simulink model "traj_generator"  (R2020b)
settings: Solver=ode45  StartTime=0.0  StopTime=1  MaxStep=0.01  RelTol=1e-3
values from neighbouring files (symbols this model uses):
  g = 9.81    [matlab.mat]
  m = 1.5    [matlab.mat]
undefined symbols (not defined in the file or in its folder): k_Y, x_dot_min
settings Model: Creator=Danil  LastModifiedBy=Danil

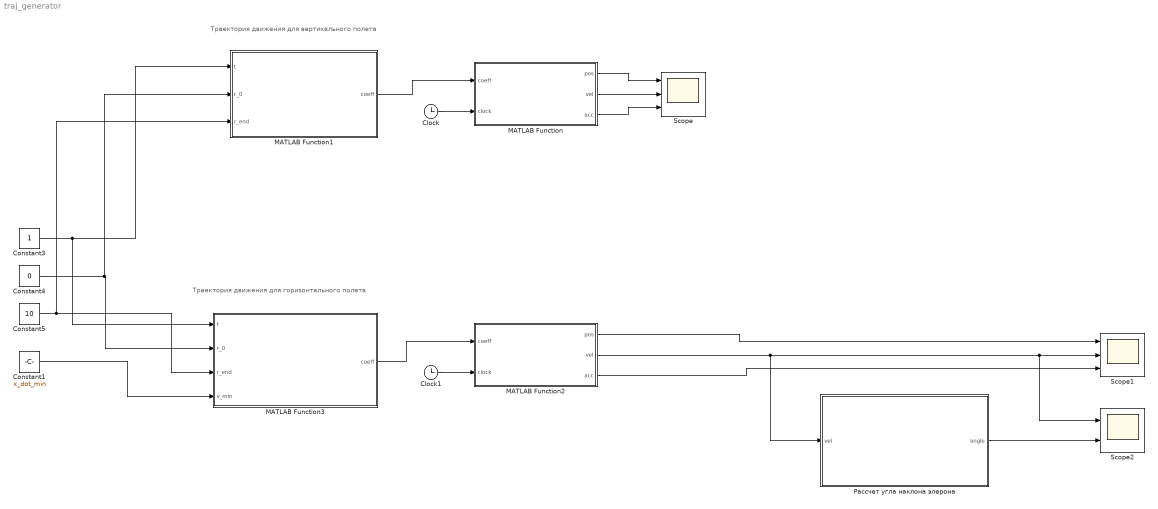
== system traj_generator ==
  note: Траектория движения для горизонтального полета
  note: Траектория движения для вертикального полета
  Clock : Clock
  Clock1 : Clock
  Constant1 : Constant  Value=x_dot_min
  Constant3 : Constant
  Constant4 : Constant  Value=0
  Constant5 : Constant  Value=10
  MATLAB Function : MATLAB Function  TreatAsAtomicUnit=on
  MATLAB Function1 : MATLAB Function  TreatAsAtomicUnit=on
  MATLAB Function2 : MATLAB Function  TreatAsAtomicUnit=on
  MATLAB Function3 : MATLAB Function  TreatAsAtomicUnit=on
  Scope : Scope  NumInputPorts=3
  Scope1 : Scope  NumInputPorts=3
  Scope2 : Scope  NumInputPorts=2
  Рассчет угла наклона элерона : Subsystem
  wires:
  Constant5/1 -> MATLAB Function1/3(r_end), MATLAB Function3/3(r_end)
  Constant4/1 -> MATLAB Function1/2(r_0), MATLAB Function3/2(r_0)
  Constant3/1 -> MATLAB Function1/1(t), MATLAB Function3/1(t)
  MATLAB Function1/1(coeff) -> MATLAB Function/1(coeff)
  Clock/1 -> MATLAB Function/2(clock)
  MATLAB Function/2(vel) -> Scope/2
  MATLAB Function/1(pos) -> Scope/1
  MATLAB Function/3(acc) -> Scope/3
  MATLAB Function2/3(acc) -> Scope1/3
  MATLAB Function2/1(pos) -> Scope1/1
  Clock1/1 -> MATLAB Function2/2(clock)
  MATLAB Function3/1(coeff) -> MATLAB Function2/1(coeff)
  Constant1/1 -> MATLAB Function3/4(v_min)
  MATLAB Function2/2(vel) -> Рассчет угла наклона элерона/1(vel), Scope2/1, Scope1/2
  Рассчет угла наклона элерона/1(angle) -> Scope2/2

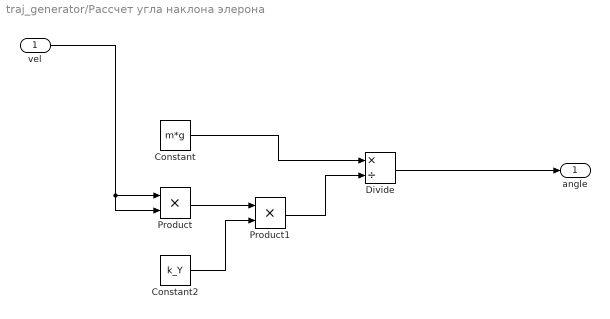
== system traj_generator/Рассчет угла наклона элерона ==
  vel : Inport
  Constant : Constant  Value=m*g
  Constant2 : Constant  Value=k_Y
  Divide : Product  Inputs=*/
  Product : Product
  Product1 : Product
  angle : Outport
  wires:
  vel/1 -> Product/2, Product/1
  Constant/1 -> Divide/1
  Constant2/1 -> Product1/2
  Divide/1 -> angle/1
  Product/1 -> Product1/1
  Product1/1 -> Divide/2

== matlab function traj_generator/MATLAB Function1 ==
  data: t input; coeff output; r_0 input; r_end input
function coeff  = calculation_coefficients(t, r_0, r_end)

x_0 = r_0;
x_dot_0 = 0;
x_ddot_0 = 0;

x_des = r_end;
x_dot_des = 0;
x_ddot_des = 0;

waypoints = [x_0    x_dot_0     x_ddot_0;
             x_des  x_dot_des   x_ddot_des]';
t = [0 t];

time_size = size(t);
n = 0;
%T = linspace(0, time_size(2) - 1, point(2));


border_conditions_sigm = reshape(waypoints(:, n + 1 : n + 2),1,[]);
%disp(border_conditions_sigm)

coeff = zeros(6, 1);

parameters = [1 * (t(n + 1) ^ 5), 1 * (t(n + 1) ^ 4), 1 * (t(n + 1) ^ 3), 1 * (t(n + 1) ^ 2), 1 * (t(n + 1) ^ 1), 1 * (t(n + 1) ^ 0);
              5 * (t(n + 1) ^ 4), 4 * (t(n + 1) ^ 3), 3 * (t(n + 1) ^ 2), 2 * (t(n + 1) ^ 1), 1 * (t(n + 1) ^ 0), 0 * (t(n + 1) ^ 0);
              20 * (t(n + 1) ^ 3), 12 * (t(n + 1) ^ 2), 6 * (t(n + 1) ^ 1), 2 * (t(n + 1) ^ 0), 0 * (t(n + 1) ^ 0), 0 * (t(n + 1) ^ 0);
              1 * (t(n + 2) ^ 5), 1 * (t(n + 2) ^ 4), 1 * (t(n + 2) ^ 3), 1 * (t(n + 2) ^ 2), 1 * (t(n + 2) ^ 1), 1 * (t(n + 2) ^ 0);
              5 * (t(n + 2) ^ 4), 4 * (t(n + 2) ^ 3), 3 * (t(n + 2) ^ 2), 2 * (t(n + 2) ^ 1), 1 * (t(n + 2) ^ 0), 0 * (t(n + 2) ^ 0);
              20 * (t(n + 2) ^ 3), 12 * (t(n + 2) ^ 2), 6 * (t(n + 2) ^ 1), 2 * (t(n + 2) ^ 0), 0 * (t(n + 2) ^ 0), 0 * (t(n + 2) ^ 0)];

coeff = inv(parameters) * border_conditions_sigm';

== matlab function traj_generator/MATLAB Function ==
  data: coeff input; pos output; clock input; vel output; acc output
function [pos, vel, acc] = trajectories_calculation(coeff, clock)

T_p = [clock^5      clock^4     clock^3     clock^2     clock   1]';
T_v = [5*clock^4    4*clock^3   3*clock^2   2*clock     1       0]';
T_a = [20*clock^3   12*clock^2  6*clock     2           0       0]';

pos = sum(coeff.*T_p);
vel = sum(coeff.*T_v);
acc = sum(coeff.*T_a);

== matlab function traj_generator/MATLAB Function2 ==
  data: coeff input; pos output; clock input; vel output; acc output
function [pos, vel, acc] = trajectories_calculation(coeff, clock)

T_p = [clock^5      clock^4     clock^3     clock^2     clock   1]';
T_v = [5*clock^4    4*clock^3   3*clock^2   2*clock     1       0]';
T_a = [20*clock^3   12*clock^2  6*clock     2           0       0]';

pos = sum(coeff.*T_p);
vel = sum(coeff.*T_v);
acc = sum(coeff.*T_a);

== matlab function traj_generator/MATLAB Function3 ==
  data: t input; coeff output; r_0 input; r_end input; v_min input
function coeff  = calculation_coefficients(t, r_0, r_end, v_min)

x_0 = r_0;
x_dot_0 = v_min;
x_ddot_0 = 0;

x_des = r_end;
x_dot_des = v_min;
x_ddot_des = 0;

waypoints = [x_0    x_dot_0     x_ddot_0;
             x_des  x_dot_des   x_ddot_des]';
t = [0 t];

time_size = size(t);
n = 0;
%T = linspace(0, time_size(2) - 1, point(2));


border_conditions_sigm = reshape(waypoints(:, n + 1 : n + 2),1,[]);
%disp(border_conditions_sigm)

coeff = zeros(6, 1);

parameters = [1 * (t(n + 1) ^ 5), 1 * (t(n + 1) ^ 4), 1 * (t(n + 1) ^ 3), 1 * (t(n + 1) ^ 2), 1 * (t(n + 1) ^ 1), 1 * (t(n + 1) ^ 0);
              5 * (t(n + 1) ^ 4), 4 * (t(n + 1) ^ 3), 3 * (t(n + 1) ^ 2), 2 * (t(n + 1) ^ 1), 1 * (t(n + 1) ^ 0), 0 * (t(n + 1) ^ 0);
              20 * (t(n + 1) ^ 3), 12 * (t(n + 1) ^ 2), 6 * (t(n + 1) ^ 1), 2 * (t(n + 1) ^ 0), 0 * (t(n + 1) ^ 0), 0 * (t(n + 1) ^ 0);
              1 * (t(n + 2) ^ 5), 1 * (t(n + 2) ^ 4), 1 * (t(n + 2) ^ 3), 1 * (t(n + 2) ^ 2), 1 * (t(n + 2) ^ 1), 1 * (t(n + 2) ^ 0);
              5 * (t(n + 2) ^ 4), 4 * (t(n + 2) ^ 3), 3 * (t(n + 2) ^ 2), 2 * (t(n + 2) ^ 1), 1 * (t(n + 2) ^ 0), 0 * (t(n + 2) ^ 0);
              20 * (t(n + 2) ^ 3), 12 * (t(n + 2) ^ 2), 6 * (t(n + 2) ^ 1), 2 * (t(n + 2) ^ 0), 0 * (t(n + 2) ^ 0), 0 * (t(n + 2) ^ 0)];

coeff = inv(parameters) * border_conditions_sigm';
